simulink subsystem "calc_rate"  (R2025b)
settings: Solver=VariableStepAuto  StartTime=0.0  StopTime=10.0  RelTol=1e-3
settings Model: Creator=kawan  LastModifiedBy=kawan

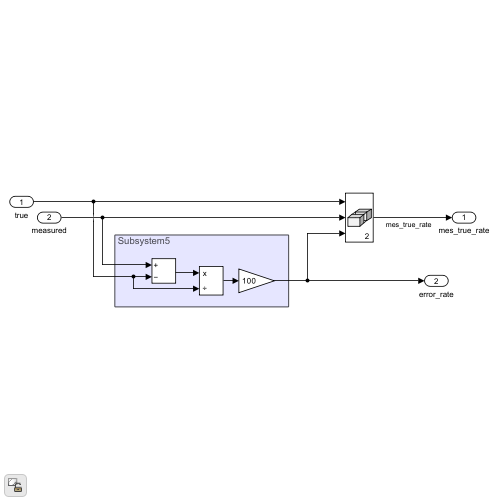
[thumbnail: Simulink's stored preview of the top-level diagram]
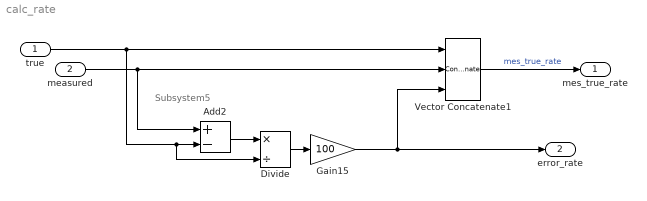
== system calc_rate ==
  note: Subsystem5
  true : Inport
  measured : Inport  Port=2
  Add2 : Sum  Inputs=+-
  Divide : Product  Inputs=*/
  Gain15 : Gain  Gain=100
  Vector Concatenate1 : Concatenate  NumInputs=3  Mode=Multidimensional array  ConcatenateDimension=2
  mes_true_rate : Outport
  error_rate : Outport  Port=2
  wires:
  Gain15/1 -> error_rate/1, Vector Concatenate1/3
  Vector Concatenate1/1 -> mes_true_rate/1  "mes_true_rate"
  measured/1 -> Vector Concatenate1/2, Add2/1
  Add2/1 -> Divide/1
  Divide/1 -> Gain15/1
  true/1 -> Vector Concatenate1/1, Divide/2, Add2/2
